simulink library "PvtLibPLAN"  (R2020b)
settings: Solver=VariableStepAuto  StartTime=0.0  StopTime=10.0  RelTol=1e-3
undefined symbols (not defined in the file): P_Global_DxvFrontBumper_m, P_Global_DxvRearBumper_m, P_VSM_DPC_HWALineRearA2Factor, P_VSM_DPC_HWALineRearA3Factor
libraries: simulink x6
settings Model: Creator=GW00166368  LastModifiedBy=GW00166368

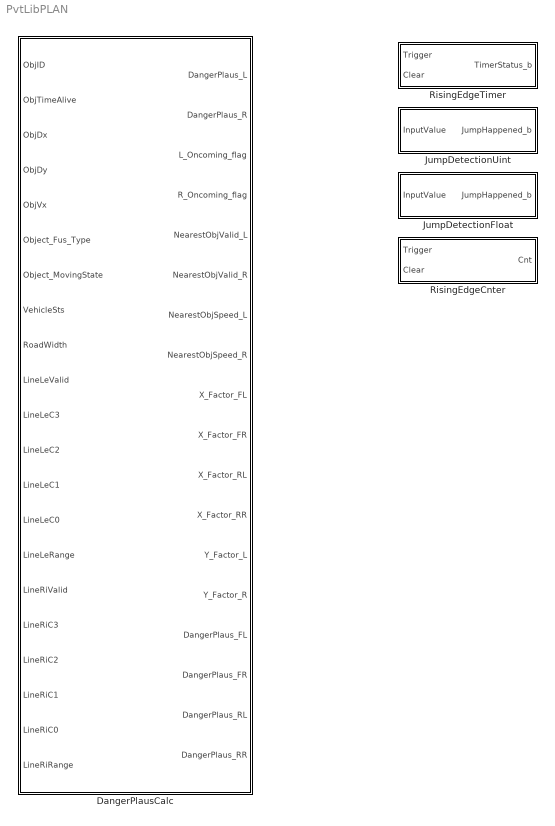
== system PvtLibPLAN ==
  DangerPlausCalc : Subsystem  TreatAsAtomicUnit=on  mask{ObjNum=1}
      mask prompts: ObjNum "目标数量"
      settings: RTWFcnNameOpts=Use subsystem name  RTWFileNameOpts=Use function name
      mask DialogControl DescGroupVar Prompt: 功能描述
      mask DialogControl DescTextVar Prompt: 计算周边目标的危险度，目标属性以数组的形式输入，目标数量>=1
      mask DialogControl ParameterGroupVar Prompt: 目标属性
  JumpDetectionFloat : Subsystem  mask(JumpDetectionFloat){StartValue=0, FinishValue=0, Tolerance=0}
      mask help: 检测一个周期内，浮点数输入是否存在从StartValue到FinishValue的跳变，允许Tolerance的误差
  JumpDetectionUint : Subsystem  mask(JumpDetectionUint){StartValue=0, FinishValue=0}
      mask help: 检测一个周期内，整形输入是否存在从StartValue到FinishValue的跳变，StartValue和FinishValue非整数时四舍五入取整。
  RisingEdgeCnter : Subsystem  mask(RisingEdgeCnter){}
      mask help: 每当rigger（Boolean）端口检测到一次上升沿后，计数一次。当Clear（Boolean）端口检测到true后，计数器清零。输出计数次数
  RisingEdgeTimer : Subsystem  mask(RisingEdgeTimer){MaxCnt=0}
      mask help: 当Trigger（Boolean）端口检测到上升沿后，开始计数，输出TimerStatus_b（Boolean）为true。当计数达到MaxCnt时，或Clear（Boolean）端口检测到true后，计数器清零。TimerStatus_b输出false。若MaxCycles==0，则只能由Clear端口输入true将输出置false。

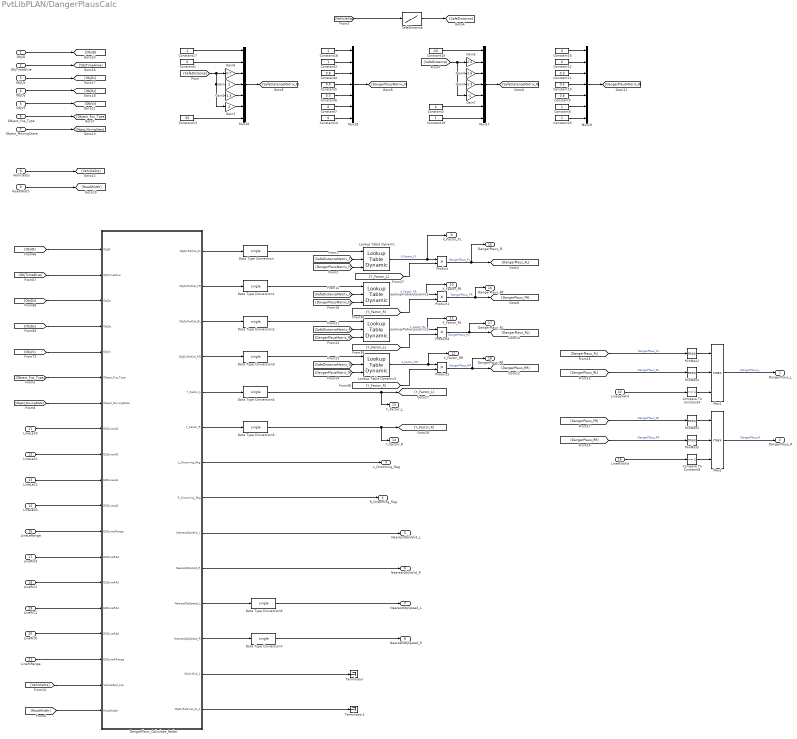
== system PvtLibPLAN/DangerPlausCalc ==
  ObjID : Inport  PortDimensions=ObjNum
  ObjTimeAlive : Inport  Port=2  PortDimensions=ObjNum
  ObjDx : Inport  Port=3  PortDimensions=ObjNum
  ObjDy : Inport  Port=4  PortDimensions=ObjNum
  ObjVx : Inport  Port=5  PortDimensions=ObjNum
  Object_Fus_Type : Inport  Port=6  PortDimensions=ObjNum
  Object_MovingState : Inport  Port=7  PortDimensions=ObjNum
  VehicleSts : Inport  Port=8
  RoadWidth : Inport  Port=9
  LineLeValid : Inport  Port=10
  LineLeC3 : Inport  Port=11
  LineLeC2 : Inport  Port=12
  LineLeC1 : Inport  Port=13
  LineLeC0 : Inport  Port=14
  LineLeRange : Inport  Port=15
  LineRiValid : Inport  Port=16
  LineRiC3 : Inport  Port=17
  LineRiC2 : Inport  Port=18
  LineRiC1 : Inport  Port=19
  LineRiC0 : Inport  Port=20
  LineRiRange : Inport  Port=21
  Compare To Constant4 : simulink/Logic and Bit Operations/Compare To Constant  relop=~=  const=1  OutDataTypeStr=uint8
  Compare To Constant9 : simulink/Logic and Bit Operations/Compare To Constant  relop=~=  const=1  OutDataTypeStr=uint8
  Constant{1..2,7,12,14,16} (6 alike) : Constant  Value=0  OutDataTypeStr=Inherit: Inherit via back propagation
  Constant10 : Constant  Value=0.5  OutDataTypeStr=Inherit: Inherit via back propagation
  Constant11 : Constant  Value=0.3  OutDataTypeStr=Inherit: Inherit via back propagation
  Constant13 : Constant  Value=50  OutDataTypeStr=Inherit: Inherit via back propagation
  Constant15 : Constant  Value=-50  OutDataTypeStr=Inherit: Inherit via back propagation
  Constant17 : Constant  Value=-1  OutDataTypeStr=Inherit: Inherit via back propagation
  Constant{3,8,18..20} (5 alike) : Constant  OutDataTypeStr=Inherit: Inherit via back propagation
  Constant4 : Constant  Value=0.8  OutDataTypeStr=Inherit: Inherit via back propagation
  Constant5 : Constant  Value=0.5  OutDataTypeStr=Inherit: Inherit via back propagation
  Constant6 : Constant  Value=0.3  OutDataTypeStr=Inherit: Inherit via back propagation
  Constant9 : Constant  Value=0.8  OutDataTypeStr=Inherit: Inherit via back propagation
  DangerPlaus_Calculate_Radar : MATLAB Function  TreatAsAtomicUnit=on
  Data Type Conversion{,1..7} (8 alike) : DataTypeConversion  OutDataTypeStr=single
  Gain : Gain
  Gain1 : Gain  Gain=1.3
  Gain2 : Gain  Gain=2
  Gain3 : Gain  Gain=-1.3
  Gain4 : Gain  Gain=-1.6
  Gain5 : Gain  Gain=-2.5
  Gain6 : Gain  Gain=0.7
  Gain7 : Gain  Gain=-1
  Lookup Table Dynamic{,1..3} (4 alike) : simulink/Lookup Tables/Lookup Table Dynamic  LookUpMeth=Interpolation-Use End Values  OutDataType=fixdt('single')  OutScaling=[]  OutputDataTypeScalingMode=Specify via dialog  OutDataTypeStr=single  DoSatur=off
  Max1 : MinMax  Function=max  Inputs=3
  Max2 : MinMax  Function=max  Inputs=3
  MinMax{2..5} (4 alike) : MinMax  Function=max
  Mux{16..19} (4 alike) : Mux  Inputs=7
  Product{,1,4..5} (4 alike) : Product
  SafeDistance : Lookup_n-D  NumberOfTableDimensions=1  BreakpointsForDimension1=[0,20,30,40,120]  Table=[4,5,8,10,10]  RndMeth=Simplest  InputSameDT=on
  Terminator : Terminator
  Terminator1 : Terminator
  DangerPlaus_L : Outport  OutDataTypeStr=single
  DangerPlaus_R : Outport  Port=2  OutDataTypeStr=single
  L_Oncoming_flag : Outport  Port=3  OutDataTypeStr=boolean
  R_Oncoming_flag : Outport  Port=4  OutDataTypeStr=boolean
  NearestObjValid_L : Outport  Port=5  OutDataTypeStr=boolean
  NearestObjValid_R : Outport  Port=6  OutDataTypeStr=boolean
  NearestObjSpeed_L : Outport  Port=7  OutDataTypeStr=single
  NearestObjSpeed_R : Outport  Port=8  OutDataTypeStr=single
  X_Factor_FL : Outport  Port=9  OutDataTypeStr=single
  X_Factor_FR : Outport  Port=10  OutDataTypeStr=single
  X_Factor_RL : Outport  Port=11  OutDataTypeStr=single
  X_Factor_RR : Outport  Port=12  OutDataTypeStr=single
  Y_Factor_L : Outport  Port=13  OutDataTypeStr=single
  Y_Factor_R : Outport  Port=14  OutDataTypeStr=single
  DangerPlaus_FL : Outport  Port=15  OutDataTypeStr=single
  DangerPlaus_FR : Outport  Port=16  OutDataTypeStr=single
  DangerPlaus_RL : Outport  Port=17  OutDataTypeStr=single
  DangerPlaus_RR : Outport  Port=18  OutDataTypeStr=single
  wires:
  ObjID/1 -> [ObjID]
  ObjTimeAlive/1 -> [ObjTimeAlive]
  ObjDx/1 -> [ObjDx]
  ObjDy/1 -> [ObjDy]
  ObjVx/1 -> [ObjVx]
  Constant20/1 -> Mux19/7
  Constant2/1 -> Mux17/6
  MinMax5/1 -> Max2/2
  Constant6/1 -> Mux18/5
  Gain2/1 -> Mux16/6
  Max1/1 -> DangerPlaus_L/1  "DangerPlaus_L"
  DangerPlaus_Calculate_Radar/1(ObjDxRelCal_FL) -> Data Type Conversion/1
  [SafeDistanceMatrix_R] -> Lookup Table Dynamic3/2
  Mux19/1 -> [DangerPlausMatrix_R]
  Constant4/1 -> Mux18/3
  Gain7/1 -> Mux17/5
  Constant19/1 -> Mux17/7
  Constant14/1 -> Mux18/7
  Constant7/1 -> Mux18/6
  Product4/1 -> DangerPlaus_RL/1, [DangerPlaus_RL]  "DangerPlaus_RL"
  [SafeDistanceMatrix_F] -> Lookup Table Dynamic1/2
  [DangerPlaus_FL] -> MinMax2/1  "DangerPlaus_FL"
  Constant5/1 -> Mux18/4
  Gain1/1 -> Mux16/5
  Constant3/1 -> Mux18/2
  [ObjDx] -> DangerPlaus_Calculate_Radar/3(ObjDx)
  Lookup Table Dynamic1/1 -> X_Factor_FR/1, Product1/1  "X_Factor_FR"
  Gain/1 -> Mux16/4
  Mux18/1 -> [DangerPlausMatrix_F]
  Constant9/1 -> Mux19/5
  Constant16/1 -> Mux19/1
  [DangerPlaus_RL] -> MinMax4/1  "DangerPlaus_RL"
  [SafeDistance] -> Gain4/1, Gain3/1, Gain7/1, Gain5/1
  LineRiValid/1 -> Compare To Constant9/1
  Mux16/1 -> [SafeDistanceMatrix_F]
  [Y_Factor_L] -> Product/2
  [Y_Factor_L] -> Product4/2
  Constant8/1 -> Mux19/6
  MinMax4/1 -> Max1/2
  MinMax2/1 -> Max1/1
  Max2/1 -> DangerPlaus_R/1  "DangerPlaus_R"
  DangerPlaus_Calculate_Radar/2(ObjDxRelCal_FR) -> Data Type Conversion1/1
  [SafeDistanceMatrix_F] -> Lookup Table Dynamic/2
  Compare To Constant9/1 -> Max2/3
  Lookup Table Dynamic3/1 -> X_Factor_RR/1, Product5/1  "X_Factor_RR"
  Compare To Constant4/1 -> Max1/3
  Lookup Table Dynamic/1 -> X_Factor_FL/1, Product/1  "X_Factor_FL"
  Gain3/1 -> Mux17/4
  [DangerPlausMatrix_R] -> Lookup Table Dynamic3/3
  DangerPlaus_Calculate_Radar/4(ObjDxRelCal_RR) -> Data Type Conversion3/1
  Gain4/1 -> Mux17/3
  [Y_Factor_R] -> Product5/2
  Constant1/1 -> Mux16/2
  Product5/1 -> DangerPlaus_RR/1, [DangerPlaus_RR]  "DangerPlaus_RR"
  [SafeDistanceMatrix_R] -> Lookup Table Dynamic2/2
  [DangerPlaus_FR] -> MinMax3/1  "DangerPlaus_FR"
  Constant13/1 -> Mux16/7
  [DangerPlausMatrix_F] -> Lookup Table Dynamic1/3
  [ObjVx] -> DangerPlaus_Calculate_Radar/5(ObjVx)
  Constant18/1 -> Mux18/1
  Lookup Table Dynamic2/1 -> X_Factor_RL/1, Product4/1  "X_Factor_RL"
  Constant10/1 -> Mux19/4
  [Y_Factor_R] -> Product1/2
  SafeDistance/1 -> [SafeDistance]
  Constant15/1 -> Mux17/1
  DangerPlaus_Calculate_Radar/3(ObjDxRelCal_RL) -> Data Type Conversion2/1
  Constant11/1 -> Mux19/3
  MinMax3/1 -> Max2/1
  Gain5/1 -> Mux17/2
  Mux17/1 -> [SafeDistanceMatrix_R]
  [ObjTimeAlive] -> DangerPlaus_Calculate_Radar/2(ObjTimeAlive)
  [ObjDy] -> DangerPlaus_Calculate_Radar/4(ObjDy)
  [DangerPlausMatrix_R] -> Lookup Table Dynamic2/3
  LineLeValid/1 -> Compare To Constant4/1
  [DangerPlaus_RR] -> MinMax5/1  "DangerPlaus_RR"
  [SafeDistance] -> Gain1/1, Gain2/1, Gain/1, Gain6/1
  Product1/1 -> DangerPlaus_FR/1, [DangerPlaus_FR]  "DangerPlaus_FR"
  [DangerPlausMatrix_F] -> Lookup Table Dynamic/3
  Gain6/1 -> Mux16/3
  Constant17/1 -> Mux16/1
  Product/1 -> DangerPlaus_FL/1, [DangerPlaus_FL]  "DangerPlaus_FL"
  [ObjID] -> DangerPlaus_Calculate_Radar/1(ObjID)
  Constant12/1 -> Mux19/2
  [VehicleSts] -> SafeDistance/1
  DangerPlaus_Calculate_Radar/9(NearestObjValid_L) -> NearestObjValid_L/1
  DangerPlaus_Calculate_Radar/10(NearestObjValid_R) -> NearestObjValid_R/1
  DangerPlaus_Calculate_Radar/11(NearestObjSpeed_L) -> Data Type Conversion6/1
  DangerPlaus_Calculate_Radar/12(NearestObjSpeed_R) -> Data Type Conversion7/1
  RoadWidth/1 -> [RoadWidth]
  DangerPlaus_Calculate_Radar/5(Y_Factor_L) -> Data Type Conversion4/1
  DangerPlaus_Calculate_Radar/6(Y_Factor_R) -> Data Type Conversion5/1
  VehicleSts/1 -> [VehicleSts]
  DangerPlaus_Calculate_Radar/13(ObjVxGnd_1) -> Terminator/1
  DangerPlaus_Calculate_Radar/14(ObjDxRelFinal_FL_1) -> Terminator1/1
  LineLeC3/1 -> DangerPlaus_Calculate_Radar/8(ESSLineLA3)
  LineLeC2/1 -> DangerPlaus_Calculate_Radar/9(ESSLineLA2)
  LineLeC1/1 -> DangerPlaus_Calculate_Radar/10(ESSLineLA1)
  LineLeC0/1 -> DangerPlaus_Calculate_Radar/11(ESSLineLA0)
  LineRiC3/1 -> DangerPlaus_Calculate_Radar/13(ESSLineRA3)
  LineRiC2/1 -> DangerPlaus_Calculate_Radar/14(ESSLineRA2)
  LineRiC1/1 -> DangerPlaus_Calculate_Radar/15(ESSLineRA1)
  LineRiC0/1 -> DangerPlaus_Calculate_Radar/16(ESSLineRA0)
  [VehicleSts] -> DangerPlaus_Calculate_Radar/18(VehicleSpd_kph)
  [RoadWidth] -> DangerPlaus_Calculate_Radar/19(RoadWidth)
  Object_Fus_Type/1 -> [Object_Fus_Type]
  Object_MovingState/1 -> [Object_MovingState]
  [Object_MovingState] -> DangerPlaus_Calculate_Radar/7(Object_MovingState)
  [Object_Fus_Type] -> DangerPlaus_Calculate_Radar/6(Object_Fus_Type)
  LineLeRange/1 -> DangerPlaus_Calculate_Radar/12(ESSLineLRange)
  LineRiRange/1 -> DangerPlaus_Calculate_Radar/17(ESSLineRRange)
  DangerPlaus_Calculate_Radar/7(L_Oncoming_flag) -> L_Oncoming_flag/1
  DangerPlaus_Calculate_Radar/8(R_Oncoming_flag) -> R_Oncoming_flag/1
  Data Type Conversion/1 -> Lookup Table Dynamic/1
  Data Type Conversion1/1 -> Lookup Table Dynamic1/1
  Data Type Conversion2/1 -> Lookup Table Dynamic2/1
  Data Type Conversion3/1 -> Lookup Table Dynamic3/1
  Data Type Conversion4/1 -> [Y_Factor_L], Y_Factor_L/1
  Data Type Conversion5/1 -> Y_Factor_R/1, [Y_Factor_R]
  Data Type Conversion6/1 -> NearestObjSpeed_L/1
  Data Type Conversion7/1 -> NearestObjSpeed_R/1

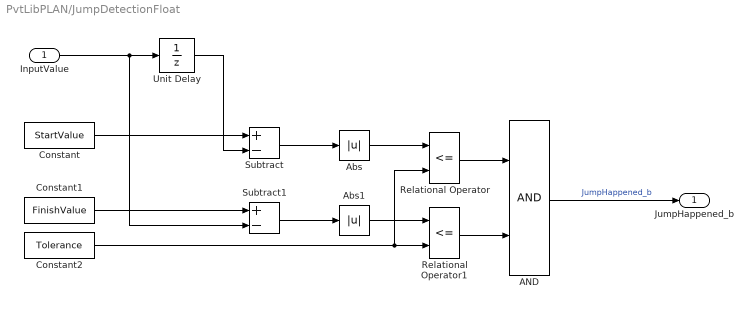
== system PvtLibPLAN/JumpDetectionFloat ==
  InputValue : Inport  OutDataTypeStr=single
  AND : Logic  AllPortsSameDT=off  OutDataTypeStr=boolean
  Abs : Abs
  Abs1 : Abs
  Constant : Constant  Value=StartValue  OutDataTypeStr=single
  Constant1 : Constant  Value=FinishValue  OutDataTypeStr=single
  Constant2 : Constant  Value=Tolerance  OutDataTypeStr=single
  Relational Operator : RelationalOperator  Operator=<=  OutDataTypeStr=boolean  RndMeth=Simplest
  Relational Operator1 : RelationalOperator  Operator=<=  OutDataTypeStr=boolean  RndMeth=Simplest
  Subtract : Sum  Inputs=+-
  Subtract1 : Sum  Inputs=+-
  Unit Delay : UnitDelay  SampleTime=-1  HasFrameUpgradeWarning=on
  JumpHappened_b : Outport
  wires:
  Unit Delay/1 -> Subtract/2
  Constant1/1 -> Subtract1/1
  Subtract1/1 -> Abs1/1
  Abs1/1 -> Relational Operator1/1
  Constant2/1 -> Relational Operator/2, Relational Operator1/2
  Abs/1 -> Relational Operator/1
  Subtract/1 -> Abs/1
  Constant/1 -> Subtract/1
  InputValue/1 -> Unit Delay/1, Subtract1/2
  Relational Operator/1 -> AND/1
  Relational Operator1/1 -> AND/2
  AND/1 -> JumpHappened_b/1  "JumpHappened_b"

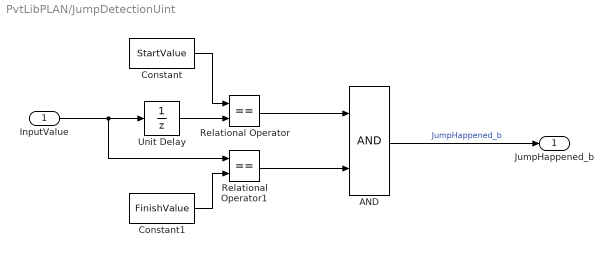
== system PvtLibPLAN/JumpDetectionUint ==
  InputValue : Inport  OutDataTypeStr=uint8
  AND : Logic  AllPortsSameDT=off  OutDataTypeStr=boolean
  Constant : Constant  Value=StartValue  OutDataTypeStr=uint8
  Constant1 : Constant  Value=FinishValue  OutDataTypeStr=uint8
  Relational Operator : RelationalOperator  Operator===  OutDataTypeStr=boolean  RndMeth=Simplest
  Relational Operator1 : RelationalOperator  Operator===  OutDataTypeStr=boolean  RndMeth=Simplest
  Unit Delay : UnitDelay  SampleTime=-1  HasFrameUpgradeWarning=on
  JumpHappened_b : Outport
  wires:
  Constant1/1 -> Relational Operator1/2
  Constant/1 -> Relational Operator/1
  AND/1 -> JumpHappened_b/1  "JumpHappened_b"
  Relational Operator1/1 -> AND/2
  Relational Operator/1 -> AND/1
  InputValue/1 -> Unit Delay/1, Relational Operator1/1
  Unit Delay/1 -> Relational Operator/2

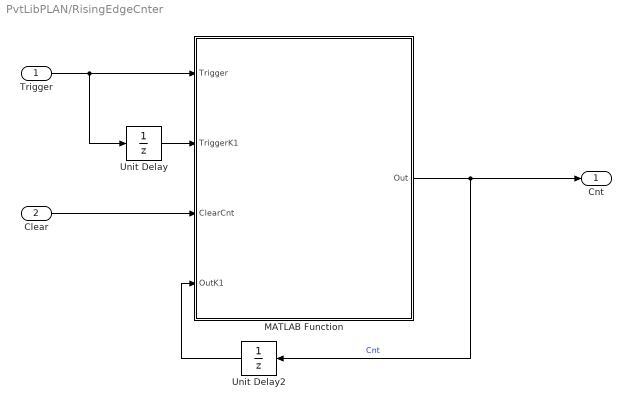
== system PvtLibPLAN/RisingEdgeCnter ==
  Trigger : Inport  OutDataTypeStr=boolean
  Clear : Inport  Port=2  OutDataTypeStr=boolean
  MATLAB Function : MATLAB Function  TreatAsAtomicUnit=on
  Unit Delay : UnitDelay  SampleTime=-1  HasFrameUpgradeWarning=on
  Unit Delay2 : UnitDelay  SampleTime=-1  HasFrameUpgradeWarning=on
  Cnt : Outport  OutDataTypeStr=uint8
  wires:
  Clear/1 -> MATLAB Function/3(ClearCnt)
  Trigger/1 -> MATLAB Function/1(Trigger), Unit Delay/1
  Unit Delay/1 -> MATLAB Function/2(TriggerK1)
  MATLAB Function/1(Out) -> Cnt/1, Unit Delay2/1  "Cnt"
  Unit Delay2/1 -> MATLAB Function/4(OutK1)

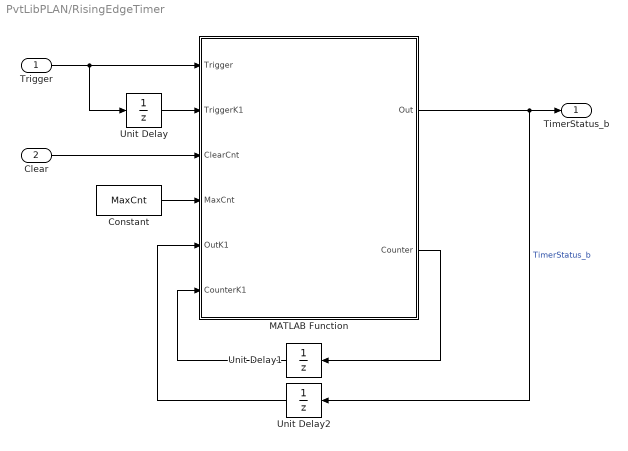
== system PvtLibPLAN/RisingEdgeTimer ==
  Trigger : Inport  OutDataTypeStr=boolean
  Clear : Inport  Port=2  OutDataTypeStr=boolean
  Constant : Constant  Value=MaxCnt  OutDataTypeStr=uint16
  MATLAB Function : MATLAB Function  TreatAsAtomicUnit=on
  Unit Delay : UnitDelay  SampleTime=-1  HasFrameUpgradeWarning=on
  Unit Delay1 : UnitDelay  SampleTime=-1  HasFrameUpgradeWarning=on
  Unit Delay2 : UnitDelay  SampleTime=-1  HasFrameUpgradeWarning=on
  TimerStatus_b : Outport  OutDataTypeStr=boolean
  wires:
  Unit Delay2/1 -> MATLAB Function/5(OutK1)
  MATLAB Function/1(Out) -> Unit Delay2/1, TimerStatus_b/1  "TimerStatus_b"
  Constant/1 -> MATLAB Function/4(MaxCnt)
  MATLAB Function/2(Counter) -> Unit Delay1/1
  Unit Delay/1 -> MATLAB Function/2(TriggerK1)
  Unit Delay1/1 -> MATLAB Function/6(CounterK1)
  Trigger/1 -> Unit Delay/1, MATLAB Function/1(Trigger)
  Clear/1 -> MATLAB Function/3(ClearCnt)

== matlab function PvtLibPLAN/DangerPlausCalc/DangerPlaus_Calculate_Radar ==
  data: ObjID input; ObjTimeAlive input; ObjDx input; ObjDxRelCal_FL output; ObjDxRelCal_FR output; ObjDxRelCal_RL output; ObjDxRelCal_RR output; ObjDy input; ObjVx input; Object_Fus_Type input; Object_MovingState input; ESSLineLA3 input; ESSLineLA2 input; ESSLineLA1 input; ESSLineLA0 input; ESSLineLRange input; ESSLineRA3 input; ESSLineRA2 input; ESSLineRA1 input; ESSLineRA0 input; ESSLineRRange input; VehicleSpd_kph input; RoadWidth input; P_VSM_DPC_HWALineRearA3Factor parameter; P_VSM_DPC_HWALineRearA2Factor parameter; P_Global_DxvFrontBumper_m parameter; Y_Factor_L output; P_Global_DxvRearBumper_m parameter; Y_Factor_R output; L_Oncoming_flag output; R_Oncoming_flag output; NearestObjValid_L output boolean; NearestObjValid_R output boolean; NearestObjSpeed_L output; NearestObjSpeed_R output; ObjVxGnd_1 output; ObjDxRelFinal_FL_1 output; ObjNum parameter
function [ObjDxRelCal_FL,ObjDxRelCal_FR,ObjDxRelCal_RL,ObjDxRelCal_RR,Y_Factor_L,Y_Factor_R,...
    L_Oncoming_flag,R_Oncoming_flag,...
    NearestObjValid_L,NearestObjValid_R,NearestObjSpeed_L,NearestObjSpeed_R, ObjVxGnd_1, ObjDxRelFinal_FL_1] = ...
    fcn(ObjID, ObjTimeAlive, ObjDx, ObjDy, ObjVx, Object_Fus_Type, Object_MovingState,...
    ESSLineLA3, ESSLineLA2,ESSLineLA1, ESSLineLA0, ESSLineLRange,...
    ESSLineRA3, ESSLineRA2,ESSLineRA1, ESSLineRA0, ESSLineRRange,...
    VehicleSpd_kph,RoadWidth,...
    P_VSM_DPC_HWALineRearA3Factor, P_VSM_DPC_HWALineRearA2Factor,...
    P_Global_DxvFrontBumper_m, P_Global_DxvRearBumper_m, ObjNum)

InvalidValue = single(999);
ObjTimeAliveCounter = 3;
TimeTurn = 4;
TimeReact = 3;
ObjDxRelCal_FL = zeros(ObjNum,1);
ObjDxRelCal_FR = zeros(ObjNum,1);
ObjDxRelCal_RL = zeros(ObjNum,1);
ObjDxRelCal_RR = zeros(ObjNum,1);
DeltaDistance_Y_L = zeros(ObjNum,1);
DeltaDistance_Y_R = zeros(ObjNum,1);
Y_Factor_L = zeros(ObjNum,1);
Y_Factor_R = zeros(ObjNum,1);
L_Oncoming = zeros(ObjNum,1);
R_Oncoming = zeros(ObjNum,1);
VehicleSpd_ms = VehicleSpd_kph / 3.6;

TimePredict_L = (abs(ESSLineLA0) / RoadWidth * TimeTurn) + TimeReact;
TimePredict_R = (abs(ESSLineRA0) / RoadWidth * TimeTurn) + TimeReact;

NearestObjValid_L = false;
NearestObjDx_L = InvalidValue;
NearestObjSpeed_L = InvalidValue;
NearestObjValid_R = false;
NearestObjDx_R = InvalidValue;
NearestObjSpeed_R = InvalidValue;

ObjVxGnd_1 = single(0);
ObjDxRelFinal_FL_1 = single(0);

for i = 1:ObjNum
    if (ObjID(i) > 0)...
            && (ObjTimeAlive(i) > ObjTimeAliveCounter)
        ObjVxGnd = ObjVx(i) + VehicleSpd_ms;
        if i == 1   %%%TEST
            ObjVxGnd_1 = ObjVxGnd;
        end
        if ObjDx(i) >= 0   %Front
            ObjDxRelCal_RL(i) = - InvalidValue;
            ObjDxRelCal_RR(i) = - InvalidValue;
            %%%X Calculate%%%
            ObjDxRelInitial_Front = ObjDx(i) - P_Global_DxvFrontBumper_m;
            ObjDxRelFinal_FL = ObjDxRelInitial_Front + (ObjVxGnd * TimePredict_L) - (VehicleSpd_ms * TimePredict_L);
            if i == 1   %%%TEST
                ObjDxRelFinal_FL_1 = ObjDxRelFinal_FL;
            end
            ObjDxRelFinal_FR = ObjDxRelInitial_Front + (ObjVxGnd * TimePredict_R) - (VehicleSpd_ms * TimePredict_R);
            if (ObjDxRelInitial_Front*ObjDxRelFinal_FL)<0   %Very Dangerous
                ObjDxRelCal_FL(i) = 0;
            else
                ObjDxRelCal_FL(i) = min(ObjDxRelInitial_Front,ObjDxRelFinal_FL);
            end
            if (ObjDxRelInitial_Front*ObjDxRelFinal_FR)<0
                ObjDxRelCal_FR(i) = 0;
            else
                ObjDxRelCal_FR(i) = min(ObjDxRelInitial_Front,ObjDxRelFinal_FR);
            end
            %%%Y Calculate%%%
            P_HWALineLFrontA3Factor = single(0);
            P_HWALineRFrontA3Factor = single(0);
            P_HWALineLFrontA2Factor = Interpol(0, 1, ESSLineLRange, 1, ESSLineLRange+20, 0.7, ESSLineLRange+40, 0, ObjDx(i));
            P_HWALineRFrontA2Factor = Interpol(0, 1, ESSLineRRange, 1, ESSLineRRange+20, 0.7, ESSLineRRange+40, 0, ObjDx(i));
            Y_L = (P_HWALineLFrontA3Factor * ESSLineLA3 * ObjDx(i) * ObjDx(i) * ObjDx(i)) + (P_HWALineLFrontA2Factor * ESSLineLA2 * ObjDx(i) * ObjDx(i)) + (ESSLineLA1 * ObjDx(i)) + ESSLineLA0;
            Y_R = (P_HWALineRFrontA3Factor * ESSLineRA3 * ObjDx(i) * ObjDx(i) * ObjDx(i)) + (P_HWALineRFrontA2Factor * ESSLineRA2 * ObjDx(i) * ObjDx(i)) + (ESSLineRA1 * ObjDx(i)) + ESSLineRA0;
            %%%SD%%%
            DeltaDistance_Y_L(i) = abs(ObjDy(i) - Y_L);
            DeltaDistance_Y_R(i) = abs(ObjDy(i) - Y_R);
            %%%Feature Of Nearest Obj Of Next Lane%%%
            if (ObjDy(i) >= (Y_L - (RoadWidth / 2))) && (ObjDy(i) <= (Y_L + (RoadWidth / 2))) && (ObjDx(i) <= NearestObjDx_L)
                NearestObjValid_L = true;
                NearestObjDx_L = ObjDx(i);
                NearestObjSpeed_L = ObjVxGnd;
                if NearestObjSpeed_L < 0
                    L_Oncoming(i) = 1;
                else
                    L_Oncoming(i) = 0;
                end
            elseif (ObjDy(i) >= (Y_R - (RoadWidth / 2))) && (ObjDy(i) <= (Y_R + (RoadWidth / 2))) && (ObjDx(i) <= NearestObjDx_R)
                NearestObjValid_R = true;
                NearestObjDx_R = ObjDx(i);
                NearestObjSpeed_R = ObjVxGnd;
                if NearestObjSpeed_R < 0
                    R_Oncoming(i) = 1;
                else
                    R_Oncoming(i) = 0;
                end
            end
        else   %Rear
            ObjDxRelCal_FL(i) = InvalidValue;
            ObjDxRelCal_FR(i) = InvalidValue;
            %%%X Calculate%%%
            ObjDxRelInitial_Rear = ObjDx(i) + P_Global_DxvRearBumper_m;
            ObjDxRelFinal_RL = ObjDxRelInitial_Rear + (ObjVxGnd * TimePredict_L) - (VehicleSpd_ms * TimePredict_L);
            ObjDxRelFinal_RR = ObjDxRelInitial_Rear + (ObjVxGnd * TimePredict_R) - (VehicleSpd_ms * TimePredict_R);
            if (ObjDxRelInitial_Rear*ObjDxRelFinal_RL)<0
                ObjDxRelCal_RL(i) = 0;
            else
                ObjDxRelCal_RL(i) = max(ObjDxRelInitial_Rear,ObjDxRelFinal_RL);
            end
            
            if (ObjDxRelInitial_Rear*ObjDxRelFinal_RR)<0
                ObjDxRelCal_RR(i) = 0;
            else
                ObjDxRelCal_RR(i) = max(ObjDxRelInitial_Rear,ObjDxRelFinal_RR);
            end
            %%%Y Calculate%%%
            Y_L = (P_VSM_DPC_HWALineRearA3Factor * ESSLineLA3 * ObjDx(i) * ObjDx(i) * ObjDx(i)) + (P_VSM_DPC_HWALineRearA2Factor * ESSLineLA2 * ObjDx(i) * ObjDx(i)) + (ESSLineLA1 * ObjDx(i)) + ESSLineLA0;
            Y_R = (P_VSM_DPC_HWALineRearA3Factor * ESSLineRA3 * ObjDx(i) * ObjDx(i) * ObjDx(i)) + (P_VSM_DPC_HWALineRearA2Factor * ESSLineRA2 * ObjDx(i) * ObjDx(i)) + (ESSLineRA1 * ObjDx(i)) + ESSLineRA0;
            %%%SD%%%
            DeltaDistance_Y_L(i) = abs(ObjDy(i) - Y_L);
            DeltaDistance_Y_R(i) = abs(ObjDy(i) - Y_R);
        end
    else
        ObjDxRelCal_FL(i) = InvalidValue;
        ObjDxRelCal_FR(i) = InvalidValue;
        ObjDxRelCal_RL(i) = - InvalidValue;
        ObjDxRelCal_RR(i) = - InvalidValue;
        DeltaDistance_Y_L(i) = InvalidValue;
        DeltaDistance_Y_R(i) = InvalidValue;
    end
    if (Object_Fus_Type(i) == 0x2) && (Object_MovingState(i) == 0x3)   %F&&Stationary
        Y_Factor_L(i) = Interpol(0, 1, 0.3*RoadWidth, 1, 0.6*RoadWidth, 0, 0.6*RoadWidth+1, 0, DeltaDistance_Y_L(i));
        Y_Factor_R(i) = Interpol(0, 1, 0.3*RoadWidth, 1, 0.6*RoadWidth, 0, 0.6*RoadWidth+1, 0, DeltaDistance_Y_R(i));
    else
        Y_Factor_L(i) = Interpol(0, 1, 0.5*RoadWidth, 1, 0.5*RoadWidth+1, 0, 0.5*RoadWidth+2, 0, DeltaDistance_Y_L(i));
        Y_Factor_R(i) = Interpol(0, 1, 0.5*RoadWidth, 1, 0.5*RoadWidth+1, 0, 0.5*RoadWidth+2, 0, DeltaDistance_Y_R(i));
    end
    L_Oncoming_flag = ismember(1,L_Oncoming);
    R_Oncoming_flag = ismember(1,R_Oncoming);
end

function Out = Interpol(x1,z1,x2,z2,x3,z3,x4,z4,In)
if In<=x1
    Out = single(z1);
elseif (In>x1)&&(In<=x2)
    Out = single(z1+ (In-x1)*(z2-z1)/(x2-x1));
elseif (In>x2)&&(In<=x3)
    Out = single(z2+ (In-x2)*(z3-z2)/(x3-x2));
elseif (In>x3)&&(In<=x4)
    Out = single(z3+ (In-x3)*(z4-z3)/(x4-x3));
else
    Out = single(z4);
end

== matlab function PvtLibPLAN/RisingEdgeTimer/MATLAB Function ==
  data: Trigger input boolean; Out output boolean; TriggerK1 input boolean; ClearCnt input boolean; MaxCnt input uint16; OutK1 input boolean; CounterK1 input uint16; Counter output uint16
function [Out,Counter] = RisingEdgeTimer(Trigger,TriggerK1, ClearCnt, MaxCnt,OutK1, CounterK1)
%#codegen
if MaxCnt~=0
    if (Trigger==1)&&(TriggerK1==0)
        Counter = MaxCnt;
    else
        Counter = max(CounterK1 - uint16(1),uint16(0));
    end 
    if ClearCnt
        Counter = uint16(0);
    end
    if Counter>0x0
        Out = true;
    else
        Out = false;
    end
else
    Counter=uint16(0);
    if (Trigger==1)&&(TriggerK1==0)
        Out=true;
    else
        Out=OutK1;
    end
    if ClearCnt
        Out=false;
    end
end

== matlab function PvtLibPLAN/RisingEdgeCnter/MATLAB Function ==
  data: Trigger input boolean; Out output uint8; TriggerK1 input boolean; ClearCnt input boolean; OutK1 input uint8
function Out  = RisingEdgeTimer(Trigger,TriggerK1, ClearCnt, OutK1)
%#codegen
    if (Trigger==1)&&(TriggerK1==0)
        Out = OutK1+1;     
    else
        Out = OutK1;
    end 
    if ClearCnt
        Out = uint8(0);
    end
end
